simulink model "FaultCheck"  (R2022b)
settings: Solver=FixedStepAuto  StartTime=0.0  StopTime=10  FixedStep=1  RelTol=1e-3
undefined symbols (not defined in the file): C_Flt_IGBTULowerTempConfirmTh_u16, C_Flt_IGBTULowerTempDiagEn_b, C_Flt_IGBTULowerTempErrCode_u16, C_Flt_IGBTULowerTempPowerCoeff, C_Flt_IGBTULowerTempRecoveryTh_u16, C_Flt_IGBTULowerTempRecTh_s32, C_Flt_IGBTULowerTempTrigTh_s32, C_Flt_IGBTUOverTempConfirmTh_u16, C_Flt_IGBTUOverTempDiagEn_b, C_Flt_IGBTUOverTempErrCode_u16, C_Flt_IGBTUOverTempRecoveryTh_u16, C_Flt_IGBTUOverTempRecTh_s32, C_Flt_IGBTUOverTempTrigTh_s32, C_Flt_IGBTVLowerTempConfirmTh_u16, C_Flt_IGBTVLowerTempDiagEn_b, C_Flt_IGBTVLowerTempErrCode_u16, C_Flt_IGBTVLowerTempPowerCoeff, C_Flt_IGBTVLowerTempRecoveryTh_u16, C_Flt_IGBTVLowerTempRecTh_s32, C_Flt_IGBTVLowerTempTrigTh_s32, C_Flt_IGBTVOverTempConfirmTh_u16, C_Flt_IGBTVOverTempDiagEn_b, C_Flt_IGBTVOverTempErrCode_u16, C_Flt_IGBTVOverTempRecoveryTh_u16, C_Flt_IGBTVOverTempRecTh_s32, C_Flt_IGBTVOverTempTrigTh_s32, C_Flt_IGBTWLowerTempConfirmTh_u16, C_Flt_IGBTWLowerTempDiagEn_b, C_Flt_IGBTWLowerTempErrCode_u16, C_Flt_IGBTWLowerTempPowerCoeff, C_Flt_IGBTWLowerTempRecoveryTh_u16, C_Flt_IGBTWLowerTempRecTh_s32, C_Flt_IGBTWLowerTempTrigTh_s32, C_Flt_IGBTWOverTempConfirmTh_u16, C_Flt_IGBTWOverTempDiagEn_b, C_Flt_IGBTWOverTempErrCode_u16, C_Flt_IGBTWOverTempRecoveryTh_u16, C_Flt_IGBTWOverTempRecTh_s32, C_Flt_IGBTWOverTempTrigTh_s32, C_Flt_IuOCConfirmTh_u16, C_Flt_IuOCDiagEn_b, C_Flt_IuOCErrCode_u16, C_Flt_IuOCNegLimit_s32, C_Flt_IuOCPosLimit_s32, C_Flt_IuOCRecoveryTh_u16, C_Flt_IuZeroDriftDiagEn_b, C_Flt_IuZeroDriftErrCode_u16, C_Flt_IvOCConfirmTh_u16, C_Flt_IvOCDiagEn_b, C_Flt_IvOCErrCode_u16, C_Flt_IvOCNegLimit_s32, C_Flt_IvOCPosLimit_s32, C_Flt_IvOCRecoveryTh_u16, C_Flt_IvZeroDriftDiagEn_b, C_Flt_IvZeroDriftErrCode_u16, C_Flt_IwOCConfirmTh_u16, C_Flt_IwOCDiagEn_b, C_Flt_IwOCErrCode_u16, C_Flt_IwOCNegLimit_s32, C_Flt_IwOCPosLimit_s32 ... (+196)
libraries: YS_UserDefined_Library x21, simulink x5
(part 1 of 11)
settings Model: Creator=25313  LastModifiedBy=ZYH
settings OptimizationCC: DefaultParameterBehavior=Inlined  EnhancedBackFolding=on  PassReuseOutputArgsAs=Individual arguments  ZeroExternalMemoryAtStartup=off  ZeroInternalMemoryAtStartup=off  OptimizeBlockOrder=speed  DifferentSizesBufferReuse=on  OptimizationCustomize=off  EfficientTunableParamExpr=on
settings DebuggingCC: ParameterTunabilityLossMsg=error
settings SFSimCC: MATLABDynamicMemAlloc=off
settings RTWCC: Description=Embedded Coder  SystemTargetFile=ert.tlc  GenCodeOnly=on  TemplateMakefile=ert_default_tmf
settings CodeAppCC: ForceParamTrailComments=on  IgnoreCustomStorageClasses=off  OperatorAnnotations=on  SimulinkDataObjDesc=on  SFDataObjDesc=on  InsertBlockDesc=on
settings ERTTargetCC: TargetLangStandard=C99 (ISO)  GenerateSampleERTMain=on  IncludeMdlTerminateFcn=off  RemoveDisableFunc=on  InlinedParameterPlacement=NonHierarchical  ERTCustomFileTemplate=example_file_process.tlc

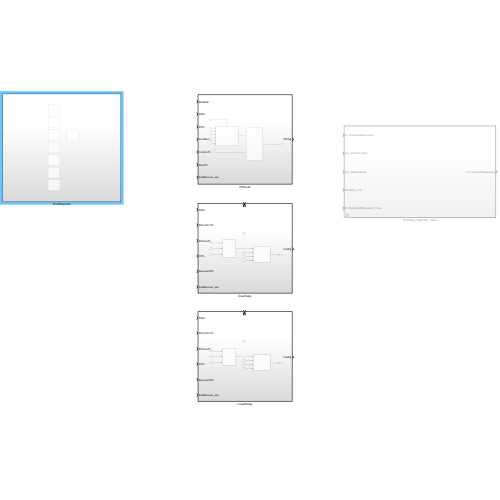
[thumbnail: Simulink's stored preview of the top-level diagram]
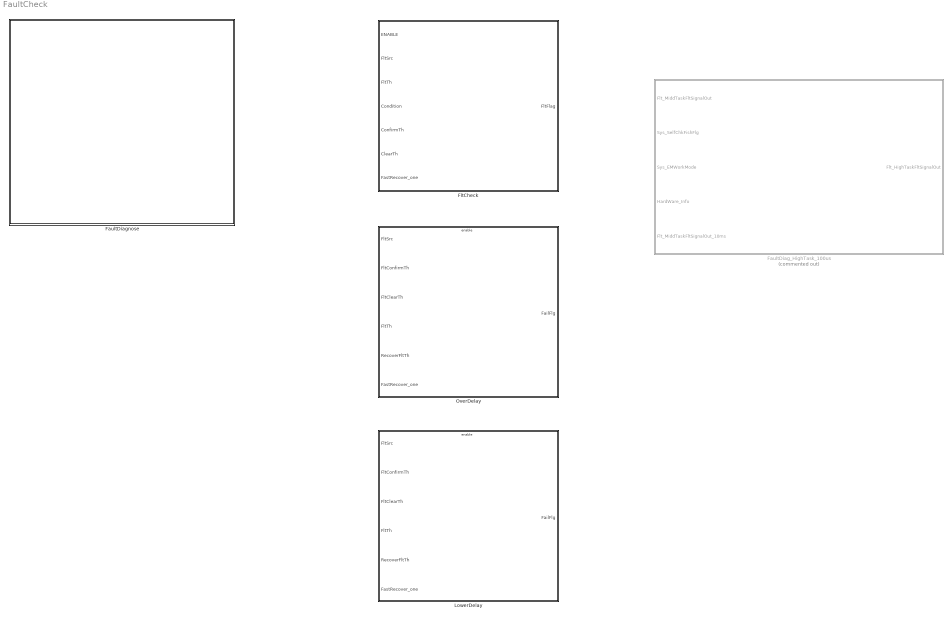
== system FaultCheck ==
  FaultDiag_HighTask_100us : Subsystem  Commented=on  TreatAsAtomicUnit=on  RTWFileName=FaultDiag_HighTask_100us_01
      settings: RTWSystemCode=Nonreusable function  RTWFcnNameOpts=Use subsystem name  RTWFileNameOpts=User specified
  FaultDiagnose : Subsystem
  FltCheck : Subsystem  TreatAsAtomicUnit=on
  LowerDelay : Subsystem
  OverDelay : Subsystem

== system FaultCheck/FaultDiag_HighTask_100us ==
  note: 其诊断主要包括：
      | 1、三相软件过流诊断
      | 2、硬件过流诊断
      | 3、电流零飘诊断
      | 4、母线电压诊断（包括一级和二级过压、欠压诊断）
      | 5、驱动电压诊断
      | 6、驱动上桥诊断
      | 7、驱动下桥诊断
      | 8、旋变电压诊断
      | 9、旋变信号诊断
      | 10、硬件电压诊断
  note: 高频故障诊断主要包括以下几个模块：
      |
      | 信号输入
      |
      | 故障诊断
      |
      | 故障收集（高频故障仲裁）
      |
      | 故障仲裁
      |
      | 信号输出
  Flt_MiddTaskFltSignalOut : Inport
  Sys_SelfChkFishFlg : Inport  Port=2
  Sys_EMWorkMode : Inport  Port=3
  HardWare_Info : Inport  Port=4
  Flt_MiddTaskFltSignalOut_10ms : Inport  Port=5
  FltDetermine : Subsystem
  FltDetn : Subsystem
  FltHandle : Subsystem
  SignalInput1 : Subsystem
  SignalOutput : Subsystem
  Flt_HighTaskFltSignalOut : Outport
  wires:
  Flt_MiddTaskFltSignalOut/1 -> SignalInput1/4(Flt_MiddTaskFltSignalOut)
  SignalInput1/1(FltSignalBus) -> FltDetn/1(FltSignalInput), [FltSignalBus]
  FltDetn/1(FltDetnOut) -> FltHandle/2(DltDetnOut)
  SignalOutput/1(Flt_HighTaskFltSignalOut) -> Flt_HighTaskFltSignalOut/1
  Sys_SelfChkFishFlg/1 -> SignalInput1/2(Sys_SelfChkFishFlg)
  Sys_EMWorkMode/1 -> SignalInput1/3(Sys_EMWorkMode)
  [FltSignalBus] -> FltHandle/1(FltSignalBus)
  FltHandle/1(FltHandleOut) -> FltDetermine/1(FltHandleOut)
  [FltSignalBus] -> FltDetermine/2(FltSignalBus)
  FltDetermine/1(FltDetermineOut) -> SignalOutput/1(FltDetermineOut)
  HardWare_Info/1 -> SignalInput1/1(HardWare_Info)
  Flt_MiddTaskFltSignalOut_10ms/1 -> SignalInput1/5(Flt_MiddTaskFltSignalOut_10ms)

== system FaultCheck/FaultDiagnose ==
  CurrZeroDriftFltDiag : Subsystem
  IGBTTempDiag : Subsystem
  MotorSpdFltDiag : Subsystem
  MotorTempDiag : Subsystem
  PCBTempDiag : Subsystem
  PhaseCurrDiag : Subsystem  TreatAsAtomicUnit=on
  UdcLowerOneDiag : Subsystem
  UdcLowerTwoDiag : Subsystem
  UdcOverOneDiag : Subsystem
  UdcOverTwoDiag : Subsystem

== system FaultCheck/FltCheck ==
  ENABLE : Inport
  FltSrc : Inport  Port=2
  FltTh : Inport  Port=3
  Condition : Inport  Port=4
  ConfirmTh : Inport  Port=5
  ClearTh : Inport  Port=6
  FastRecover_one : Inport  Port=7
  Chart : Stateflow chart  TreatAsAtomicUnit=on
  Determination : Subsystem
  FltFlag : Outport
  wires:
  Chart/1(FltFlag) -> FltFlag/1
  FltSrc/1 -> Determination/1(FltSrc)
  FastRecover_one/1 -> Chart/2(FastRecover_one), Determination/6(FastRecover_one)
  Determination/1(FltConfirmed) -> Chart/1(FltConfirmed)
  ConfirmTh/1 -> Determination/4(ConfirmTh)
  ENABLE/1 -> Determination/Enable
  ClearTh/1 -> Determination/5(ClearTh)
  FltTh/1 -> Determination/2(FltTh)
  Condition/1 -> Determination/3(Condition)

== system FaultCheck/LowerDelay ==
  FltSrc : Inport
  FltConfirmTh : Inport  Port=2
  FltClearTh : Inport  Port=3
  FltTh : Inport  Port=4
  RecoverFltTh : Inport  Port=5
  FastRecover_one : Inport  Port=6
  Enable : EnablePort
  Hysteresis : Subsystem
  Relay : Subsystem
  FailFlg : Outport
  wires:
  FltTh/1 -> Relay/2(FltTh)
  Hysteresis/1(Out) -> FailFlg/1
  RecoverFltTh/1 -> Relay/3(RecoverFltTh)
  FastRecover_one/1 -> Hysteresis/4(FastRecover_one)
  FltSrc/1 -> Relay/1(FltSrc)
  FltClearTh/1 -> Hysteresis/3(ClearTh)
  Relay/1(Fail) -> Hysteresis/1(Fail)
  FltConfirmTh/1 -> Hysteresis/2(ConfirmTh)

== system FaultCheck/OverDelay ==
  FltSrc : Inport
  FltConfirmTh : Inport  Port=2
  FltClearTh : Inport  Port=3
  FltTh : Inport  Port=4
  RecoverFltTh : Inport  Port=5
  FastRecover_one : Inport  Port=6
  Enable : EnablePort
  Hysteresis : Subsystem
  Relay : Subsystem
  FailFlg : Outport
  wires:
  FltConfirmTh/1 -> Hysteresis/2(ConfirmTh)
  Relay/1(Fail) -> Hysteresis/1(Fail)
  FltClearTh/1 -> Hysteresis/3(ClearTh)
  FltSrc/1 -> Relay/1(FltSrc)
  FastRecover_one/1 -> Hysteresis/4(FastRecover_one)
  RecoverFltTh/1 -> Relay/3(RecoverFltTh)
  Hysteresis/1(Out) -> FailFlg/1
  FltTh/1 -> Relay/2(FltTh)

== system FaultCheck/FaultDiag_HighTask_100us/FltDetermine ==
  note: 整个故障诊断的仲裁模块，选择高频，中频和低频三种故障诊断周期的最大故障等级，最小降功率系数输出
  FltHandleOut : Inport
  FltSignalBus : Inport  Port=2
  Bus Creator : BusCreator  Inputs=4
  Bus Selector : BusSelector  OutputSignals=Flt_HighTaskFltSignalOut.Flt_HighTaskFltLvlOut_100us,Flt_HighTaskFltSignalOut.Flt_HighTaskPowRecCoef_100us
  Bus Selector1 : BusSelector  OutputSignals=Flt_FltLvlOut_1ms,Flt_PowRecCoef_1ms,Flt_MiddTaskFltLvl_10ms,Flt_MiddTaskPowRecCoef_10ms
  FliLvlOut : Subsystem
  PowRecCoefOut : Subsystem
  Subsystem1 : Subsystem
  FltDetermineOut : Outport
  wires:
  FliLvlOut/1(Flt_FltLvlOut) -> [Flt_FltLvlOut], Bus Creator/2  "Flt_FltLvlOut"
  PowRecCoefOut/1(Flt_PowRecCoef) -> Bus Creator/3  "Flt_PowRecCoefOut"
  Subsystem1/1(Flt_SwtForFOC) -> Bus Creator/4  "Flt_SwtForFOC"
  FltHandleOut/1 -> Bus Selector/1, [FltHandleOut]
  FltSignalBus/1 -> Bus Selector1/1
  Bus Creator/1 -> FltDetermineOut/1
  Bus Selector/1 -> [Flt_HighTaskFltLvlOut]  "<Flt_HighTaskFltLvlOut_100us>"
  Bus Selector/2 -> [Flt_HighTaskPowRecCoef]  "<Flt_HighTaskPowRecCoef_100us>"
  Bus Selector1/1 -> [Flt_MiddTaskFltLvlOut]  "<Flt_FltLvlOut_1ms>"
  Bus Selector1/2 -> [Flt_MiddTaskPowRecCoef]  "<Flt_PowRecCoef_1ms>"
  [Flt_HighTaskFltLvlOut] -> FliLvlOut/1(Flt_HighTaskFltLvlOut)
  [Flt_LowTaskFltLvlOut] -> FliLvlOut/3(Flt_LowTaskFltLvlOut)
  [Flt_LowTaskPowRecCoef] -> PowRecCoefOut/3(Flt_LowTaskPowRecCoef)
  [Flt_FltLvlOut] -> Subsystem1/1(Flt_FltLvlOut)
  [FltHandleOut] -> Bus Creator/1  "FltHandleOut"
  [Flt_HighTaskPowRecCoef] -> PowRecCoefOut/1(Flt_HighTaskPowRecCoef)
  Bus Selector1/4 -> [Flt_LowTaskPowRecCoef]  "<Flt_MiddTaskPowRecCoef_10ms>"
  Bus Selector1/3 -> [Flt_LowTaskFltLvlOut]  "<Flt_MiddTaskFltLvl_10ms>"
  [Flt_MiddTaskFltLvlOut] -> FliLvlOut/2(Flt_MiddTaskFltLvlOut)
  [Flt_MiddTaskPowRecCoef] -> PowRecCoefOut/2(Flt_MiddTaskPowRecCoef)

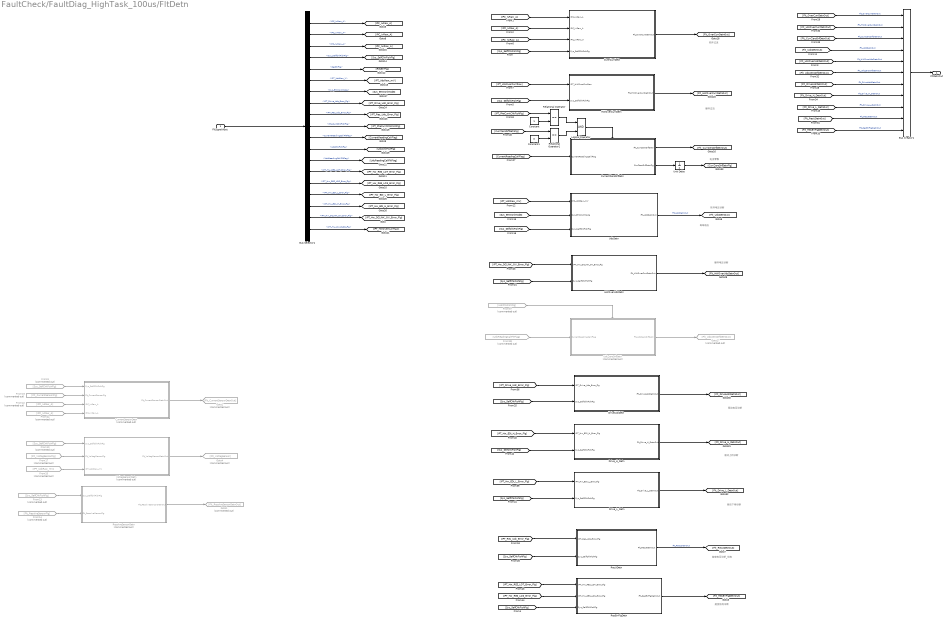
== system FaultCheck/FaultDiag_HighTask_100us/FltDetn ==
  note: 软件过流
  note: 旋变信号诊断
  note: 母线电压
  note: 旋变电压诊断_供电
  note: 硬件过流
  note: 电流零飘
  note: 软件电压诊断
  note: 硬件电压诊断
  note: 驱动电压诊断
  note: 驱动上桥诊断
  note: 驱动下桥诊断
  FltSignalInput : Inport
  Bus Creator1 : BusCreator  Inputs=11
  Bus Selector1 : BusSelector  OutputSignals=IPC_IuRaw_A,IPC_IvRaw_A,IPC_IwRaw_A,Sys_SelfChkFishFlg,ResErrFlg,IPT_UdcRaw_V,Sys_EMWorkMode,HardwareFault_Info.IPT_Drive_Udc_Error_Flg,HardwareFault_Info.IPT_Res_Udc_Error_Flg,HardwareFault_Info.PhaCurrtChkFishFlg,HardwareFault_Info.CurrentReadingCaliFltFlag,HardwareFault_Info.UdcChkFishFlg,HardwareFault_Info.UdcReadingCaliFltFlag,HardwareFault_Info.IPT_Hw_RES_LOT_Error_Flg,HardwareFault_Info.IPT_Hw_RES_LOS_Error_Flg,HardwareFault_Info.IPT_Hw_EDI_L_Error_Flg,HardwareFault_Info.IPT_Hw_EDI_H_Error_Flg,HardwareFault_Info.IPT_Hw_DCLINK_OV_Error_Flg,HardwareFault_Info.IPT_Hw_OV_CURR_Flg
  Constant : Constant  OutDataTypeStr=uint8
  Constant1 : Constant  Value=0  OutDataTypeStr=uint8
  CurrentSensorDetn : Subsystem  Commented=on
  CurrentZeroDrfDetn : Subsystem
  DriveUdcDetn : Subsystem
  Drive_H_Detn : Subsystem
  Drive_L_Detn : Subsystem
  From10 : From  Commented=on  GotoTag=Sys_SelfChkFishFlg
  From13 : From  Commented=on  GotoTag=Sys_SelfChkFishFlg
  From14 : From  Commented=on  GotoTag=Flt_ResolveSensorFlg
  From17 : From  Commented=on  GotoTag=Flt_VoltagSensorFlg
  From19 : From  Commented=on  GotoTag=Flt_CurrentSensorFlg
  From20 : From  Commented=on  GotoTag=IPT_UdcRaw_mV
  From22 : From  Commented=on  GotoTag=IPC_IuRaw_A
  From24 : From  Commented=on  GotoTag=IPC_IvRaw_A
  From37 : From  Commented=on  GotoTag=UdcChkFishFlg
  From38 : From  Commented=on  GotoTag=UdcReadingCaliFltFlag
  From9 : From  Commented=on  GotoTag=Sys_SelfChkFishFlg
  Goto1 : Goto  Commented=on  GotoTag=Flt_ResolveSensorDetnOut
  Goto2 : Goto  Commented=on  GotoTag=Flt_CurrentSensorDetnOut
  Goto27 : Goto  Commented=on  GotoTag=Flt_UdcZeroDrfDetnOut
  Goto4 : Goto  Commented=on  GotoTag=Flt_VoltagSensor
  HWOverCurrDetn : Subsystem
  HWOverUdcDetn : Subsystem
  Logical Operator : Logic  AllPortsSameDT=off  OutDataTypeStr=boolean
  OverCurrDetn : Subsystem
  RecUDetn : Subsystem
  Relational Operator : RelationalOperator  Operator===  OutDataTypeStr=boolean  RndMeth=Simplest  InputSameDT=off
  Relational Operator1 : RelationalOperator  Operator===  OutDataTypeStr=boolean  RndMeth=Simplest  InputSameDT=off
  ResErrFlgDetn : Subsystem
  ResolveSensorDetn : Subsystem  Commented=on
  UdcDetn : Subsystem
  UdcZeroDrfDetn : Subsystem  Commented=on
  Unit Delay : UnitDelay  SampleTime=-1  HasFrameUpgradeWarning=on
  VoltagSensorDetn : Subsystem  Commented=on
  FltDetnOut : Outport
  wires:
  [Sys_SelfChkFishFlg] -> OverCurrDetn/4(Sys_SelfChkFishFlg)
  [IPC_IuRaw_A] -> OverCurrDetn/1(IPC_IuRaw_A)
  [IPC_IvRaw_A] -> OverCurrDetn/2(IPC_IvRaw_A)
  OverCurrDetn/1(Flt_OverCurrDetnOut) -> [Flt_OverCurrDetnOut]
  [IPT_HWOverCurrRaw] -> HWOverCurrDetn/1(IPT_HWOverCurrRaw)
  HWOverCurrDetn/1(Flt_HWOverCurrDetnOut) -> [Flt_HWOverCurrDetnOut]
  [CurrentReadingCaliFlag] -> CurrentZeroDrfDetn/1(CurrentReadingCaliFlag)
  CurrentZeroDrfDetn/1(Flt_CurrZeroDrfDetn) -> [Flt_CurrZeroDrfDetnOut]
  [IPT_Hw_RES_LOT_Error_Flg] -> ResErrFlgDetn/1(IPT_Hw_RES_LOT_Error_Flg)
  [Sys_SelfChkFishFlg] -> ResErrFlgDetn/3(Sys_SelfChkFishFlg)
  [Sys_SelfChkFishFlg] -> HWOverCurrDetn/2(Sys_SelfChkFishFlg)
  ResErrFlgDetn/1(Flt_ResErrFlgDetnOut) -> [Flt_ResErrFlgDetnOut]
  FltSignalInput/1 -> Bus Selector1/1
  Bus Selector1/5 -> [ResErrFlg]  "<ResErrFlg>"
  Bus Selector1/2 -> [IPC_IvRaw_A]  "<IPC_IvRaw_A>"
  Bus Selector1/4 -> [Sys_SelfChkFishFlg]  "<Sys_SelfChkFishFlg>"
  Bus Selector1/17 -> [IPT_Hw_EDI_H_Error_Flg]  "<IPT_Hw_EDI_H_Error_Flg>"
  Bus Selector1/18 -> [IPT_Hw_DCLINK_OV_Error_Flg]  "<IPT_Hw_DCLINK_OV_Error_Flg>"
  Bus Selector1/6 -> [IPT_UdcRaw_mV]  "<IPT_UdcRaw_V>"
  Bus Selector1/1 -> [IPC_IuRaw_A]  "<IPC_IuRaw_A>"
  [Sys_EMWorkMode] -> UdcDetn/2(Sys_EMWorkMode)
  From13/1 -> ResolveSensorDetn/1(Sys_SelfChkFishFlg)
  From14/1 -> ResolveSensorDetn/2(Flt_ResolveSensorFlg)
  [IPT_UdcRaw_mV] -> UdcDetn/1(IPC_UdcRaw_mV)
  [IPT_Res_Udc_Error_Flg] -> RecUDetn/1(IPT_Res_Udc_Error_Flg)
  From19/1 -> CurrentSensorDetn/2(Flt_CurrentSensorFlg)
  From22/1 -> CurrentSensorDetn/3(IPC_IuRaw_A)
  VoltagSensorDetn/1(Flt_VoltagSensorDetnOut) -> Goto4/1
  From9/1 -> CurrentSensorDetn/1(Sys_SelfChkFishFlg)
  From20/1 -> VoltagSensorDetn/3(IPT_UdcRaw_mV)
  [Sys_SelfChkFishFlg] -> RecUDetn/2(Sys_SelfChkFishFlg)
  CurrentSensorDetn/1(Flt_CurrentSensorDetnOut) -> Goto2/1
  From10/1 -> VoltagSensorDetn/1(Sys_SelfChkFishFlg)
  RecUDetn/1(Flt_RecUDetnOut) -> [Flt_RecUDetnOut]  "Flt_RecUDetnOut"
  From24/1 -> CurrentSensorDetn/4(IPC_IvRaw_A)
  From17/1 -> VoltagSensorDetn/2(Flt_VoltagSensorFlg)
  [Sys_SelfChkFishFlg] -> UdcDetn/3(Sys_SelfChkFishFlg)
  UdcDetn/1(Flt_UdcDetnOut) -> [Flt_UdcDetnOut]  "Flt_UdcDetnOut"
  ResolveSensorDetn/1(Flt_ResolveSensorDetnOut) -> Goto1/1
  [Flt_RecUDetnOut] -> Bus Creator1/10  "Flt_RecUDetnOut"
  Bus Creator1/1 -> FltDetnOut/1
  [Flt_ResErrFlgDetnOut] -> Bus Creator1/11  "Flt_ResErrFlgDetnOut"
  [Flt_HWOverCurrDetnOut] -> Bus Creator1/2  "Flt_HWOverCurrDetnOut"
  [Flt_UdcDetnOut] -> Bus Creator1/4  "Flt_UdcDetnOut"
  [Flt_CurrZeroDrfDetnOut] -> Bus Creator1/3  "Flt_CurrZeroDrfDetnOut"
  [Flt_OverCurrDetnOut] -> Bus Creator1/1  "Flt_OverCurrDetnOut"
  Bus Selector1/3 -> [IPC_IwRaw_A]  "<IPC_IwRaw_A>"
  [IPC_IwRaw_A] -> OverCurrDetn/3(IPC_IwRaw_A)
  Bus Selector1/7 -> [Sys_EMWorkMode]  "<Sys_EMWorkMode>"
  Bus Selector1/8 -> [IPT_Drive_Udc_Error_Flg]  "<IPT_Drive_Udc_Error_Flg>"
  Bus Selector1/9 -> [IPT_Res_Udc_Error_Flg]  "<IPT_Res_Udc_Error_Flg>"
  Bus Selector1/11 -> [CurrentReadingCaliFlag]  "<CurrentReadingCaliFltFlag>"
  Bus Selector1/13 -> [UdcReadingCaliFltFlag]  "<UdcReadingCaliFltFlag>"
  Bus Selector1/14 -> [IPT_Hw_RES_LOT_Error_Flg]  "<IPT_Hw_RES_LOT_Error_Flg>"
  Bus Selector1/15 -> [IPT_Hw_RES_LOS_Error_Flg]  "<IPT_Hw_RES_LOS_Error_Flg>"
  Bus Selector1/16 -> [IPT_Hw_EDI_L_Error_Flg]  "<IPT_Hw_EDI_L_Error_Flg>"
  Bus Selector1/19 -> [IPT_HWOverCurrRaw]  "<IPT_Hw_OV_CURR_Flg>"
  [Sys_SelfChkFishFlg] -> HWOverUdcDetn/2(Sys_SelfChkFishFlg)
  [IPT_Hw_DCLINK_OV_Error_Flg] -> HWOverUdcDetn/1(IPT_Hw_DCLINK_OV_Error_Flg)
  UdcZeroDrfDetn/1(Flt_UdcZeroDrfDetn) -> Goto27/1
  From38/1 -> UdcZeroDrfDetn/1(CurrentReadingCaliFlag)
  From37/1 -> UdcZeroDrfDetn/Trigger
  HWOverUdcDetn/1(Flt_HWOverCurrDetnOut) -> [Flt_HWOverUdcDetnOut]
  Bus Selector1/10 -> [IPT_PhaCurrtChkFishFlg]  "<PhaCurrtChkFishFlg>"
  Bus Selector1/12 -> [UdcChkFishFlg]  "<UdcChkFishFlg>"
  DriveUdcDetn/1(Flt_DriveUdcDetnOut) -> [Flt_DriveUdcDetnOut]
  [IPT_Drive_Udc_Error_Flg] -> DriveUdcDetn/1(IPT_Drive_Udc_Error_Flg)
  [Sys_SelfChkFishFlg] -> DriveUdcDetn/2(Sys_SelfChkFishFlg)
  [IPT_Hw_EDI_L_Error_Flg] -> Drive_L_Detn/1(IPT_Hw_EDI_L_Error_Flg)
  [IPT_Hw_EDI_H_Error_Flg] -> Drive_H_Detn/1(IPT_Hw_EDI_H_Error_Flg)
  [Sys_SelfChkFishFlg] -> Drive_H_Detn/2(Sys_SelfChkFishFlg)
  [Sys_SelfChkFishFlg] -> Drive_L_Detn/2(Sys_SelfChkFishFlg)
  [IPT_Hw_RES_LOS_Error_Flg] -> ResErrFlgDetn/2(IPT_Hw_RES_LOS_Error_Flg)
  [Flt_HWOverUdcDetnOut] -> Bus Creator1/5  "Flt_HWOverUdcDetnOut"
  [Flt_UdcZeroDrfDetnOut] -> Bus Creator1/6  "Flt_UdcZeroDrfDetnOut"
  Drive_L_Detn/1(Flt_Drive_L_DetnOut) -> [Flt_Drive_L_DetnOut]
  Drive_H_Detn/1(Flt_Drive_H_DetnOut) -> [Flt_Drive_H_DetnOut]
  [Flt_DriveUdcDetnOut] -> Bus Creator1/7  "Flt_DriveUdcDetnOut"
  [Flt_Drive_H_DetnOut] -> Bus Creator1/8  "Flt_Drive_H_DetnOut"
  [Flt_Drive_L_DetnOut] -> Bus Creator1/9  "Flt_Drive_L_DetnOut"
  CurrentZeroDrfDetn/2(CurrZeroDrfDetnFlg) -> Unit Delay/1
  [IPT_PhaCurrtChkFishFlg] -> Relational Operator/1
  Relational Operator/1 -> Logical Operator/1
  [CurrZeroDrfDetnFlg] -> Relational Operator1/1
  Constant/1 -> Relational Operator/2
  Constant1/1 -> Relational Operator1/2
  Relational Operator1/1 -> Logical Operator/2
  Logical Operator/1 -> CurrentZeroDrfDetn/Enable
  Unit Delay/1 -> [CurrZeroDrfDetnFlg]

== system FaultCheck/FaultDiag_HighTask_100us/FltHandle ==
  note: 中频故障诊断的故障仲裁部分，选择故障等级最高的和故障降功率系数最低的输出，以应付多故障同时发生的情况
  FltSignalBus : Inport
  DltDetnOut : Inport  Port=2
  Bus Creator : BusCreator  Inputs=2
  Bus Creator1 : BusCreator  Inputs=3
  Bus Creator2 : BusCreator  Inputs=2
  FltLvl : Subsystem
  PowRecCoef : Subsystem
  ValOut : Subsystem
  FltHandleOut : Outport
  wires:
  Bus Creator/1 -> Bus Creator2/2  "Flt_HighTaskFltSignalOut"
  DltDetnOut/1 -> PowRecCoef/1(FltDetnIn), FltLvl/1(FltDetnIn)
  FltLvl/1(Flt_HighTaskFltLvlOut) -> Bus Creator/1  "Flt_HighTaskFltLvlOut_100us"
  PowRecCoef/1(Flt_HighTaskPowRecCoef) -> Bus Creator/2  "Flt_HighTaskPowRecCoef_100us"
  FltSignalBus/1 -> ValOut/1(FltSignalBus)
  ValOut/1(Flt_IuOut_A) -> Bus Creator1/1  "IPC_IuRaw_A"
  ValOut/2(Flt_IvOut_A) -> Bus Creator1/2  "IPC_IvRaw_A"
  Bus Creator2/1 -> FltHandleOut/1
  Bus Creator1/1 -> Bus Creator2/1  "Flt_HighTaskSignalOut"
  ValOut/3(Flt_IwOut_A) -> Bus Creator1/3  "IPC_IwRaw_A"

== system FaultCheck/FaultDiag_HighTask_100us/SignalInput1 ==
  HardWare_Info : Inport
  Sys_SelfChkFishFlg : Inport  Port=2
  Sys_EMWorkMode : Inport  Port=3
  Flt_MiddTaskFltSignalOut : Inport  Port=4
  Flt_MiddTaskFltSignalOut_10ms : Inport  Port=5
  Bus Creator : BusCreator  Inputs=14
  Bus Selector : BusSelector  OutputSignals=IPT_IRaw_A.IPC_IuRaw_A,IPT_IRaw_A.IPC_IvRaw_A,IPT_IRaw_A.IPC_IwRaw_A,ResErrFlg,IPT_TempRaw_degC.IPT_PCBTempRaw_degC,IPT_TempRaw_degC.IPT_MotorTempLow_degC_Meas,IPT_UdcRaw_V,HardwareFault_Info
  Bus Selector1 : BusSelector  OutputSignals=Flt_PowRecCoef_1ms,Flt_FltLvlOut_1ms
  Bus Selector2 : BusSelector  OutputSignals=Flt_MiddTaskFltLvl_10ms,Flt_MiddTaskPowRecCoef_10ms
  FltSignalBus : Outport
  wires:
  Bus Selector1/2 -> Bus Creator/12  "<Flt_FltLvlOut_1ms>"
  Bus Selector1/1 -> Bus Creator/11  "<Flt_PowRecCoef_1ms>"
  Sys_EMWorkMode/1 -> Bus Creator/10  "Sys_EMWorkMode"
  Sys_SelfChkFishFlg/1 -> Bus Creator/9  "Sys_SelfChkFishFlg"
  Flt_MiddTaskFltSignalOut/1 -> Bus Selector1/1
  HardWare_Info/1 -> Bus Selector/1
  Bus Creator/1 -> FltSignalBus/1
  Flt_MiddTaskFltSignalOut_10ms/1 -> Bus Selector2/1
  Bus Selector2/1 -> Bus Creator/13  "<Flt_MiddTaskFltLvl_10ms>"
  Bus Selector2/2 -> Bus Creator/14  "<Flt_MiddTaskPowRecCoef_10ms>"
  Bus Selector/1 -> Bus Creator/1  "<IPC_IuRaw_A>"
  Bus Selector/2 -> Bus Creator/2  "<IPC_IvRaw_A>"
  Bus Selector/3 -> Bus Creator/3  "<IPC_IwRaw_A>"
  Bus Selector/4 -> Bus Creator/4  "<ResErrFlg>"
  Bus Selector/5 -> Bus Creator/5  "<IPT_PCBTempRaw_degC>"
  Bus Selector/6 -> Bus Creator/6  "<IPT_MotorTempLow_degC_Meas>"
  Bus Selector/7 -> Bus Creator/7  "<IPT_UdcRaw_V>"
  Bus Selector/8 -> Bus Creator/8  "<HardwareFault_Info>"

== system FaultCheck/FaultDiag_HighTask_100us/SignalOutput ==
  FltDetermineOut : Inport
  Bus Creator : BusCreator  Inputs=6
  Bus Selector : BusSelector  OutputSignals=FltHandleOut.Flt_HighTaskSignalOut.IPC_IuRaw_A,FltHandleOut.Flt_HighTaskSignalOut.IPC_IvRaw_A,FltHandleOut.Flt_HighTaskSignalOut.IPC_IwRaw_A,Flt_PowRecCoefOut,Flt_FltLvlOut,Flt_SwtForFOC
  Constant : Constant  OutDataTypeStr=uint8
  Gain{,1..2,4} (4 alike) : Gain  OutDataTypeStr=single
  Product : Product  OutDataTypeStr=uint8
  Flt_HighTaskFltSignalOut : Outport
  wires:
  Bus Creator/1 -> Flt_HighTaskFltSignalOut/1
  FltDetermineOut/1 -> Bus Selector/1
  Bus Selector/1 -> Gain/1  "<IPC_IuRaw_A>"
  Bus Selector/2 -> Gain1/1  "<IPC_IvRaw_A>"
  Bus Selector/4 -> Gain2/1  "<Flt_PowRecCoefOut>"
  Bus Selector/6 -> Bus Creator/6  "<Flt_SwtForFOC>"
  Gain/1 -> Bus Creator/1  "IPC_luRaw_A1"
  Gain1/1 -> Bus Creator/2  "IPC_IvRaw_A1"
  Gain2/1 -> Bus Creator/4  "Flt_PowRecCoefOut1"
  Bus Selector/3 -> Gain4/1  "<IPC_IwRaw_A>"
  Gain4/1 -> Bus Creator/3  "IPC_IwRaw_A1"
  Bus Selector/5 -> Product/1  "<Flt_FltLvlOut>"
  Product/1 -> Bus Creator/5  "Flt_FltLvlOut1"
  Constant/1 -> Product/2

== system FaultCheck/FaultDiagnose/CurrZeroDriftFltDiag ==
  SysSelfCheckDownFlg : Inport
  IuZeroDriftFltFlg : Inport  Port=2
  IvZeroDriftFltFlg : Inport  Port=3
  IwZeroDriftFltFlg : Inport  Port=4
  Bus Creator : BusCreator  Inputs=3
  IuZeroDriftDiag : Subsystem
  IvZeroDriftDiag : Subsystem
  IwZeroDriftDiag : Subsystem
  Logical Operator : Logic  Operator=NOT  AllPortsSameDT=off  OutDataTypeStr=boolean
  Logical Operator1 : Logic  Operator=NOT  AllPortsSameDT=off  OutDataTypeStr=boolean
  Logical Operator2 : Logic  Operator=NOT  AllPortsSameDT=off  OutDataTypeStr=boolean
  Unit Delay : UnitDelay  SampleTime=-1  HasFrameUpgradeWarning=on
  Unit Delay1 : UnitDelay  SampleTime=-1  HasFrameUpgradeWarning=on
  Unit Delay2 : UnitDelay  SampleTime=-1  HasFrameUpgradeWarning=on
  PhaseCurrZeroDriftFltInfo : Outport
  wires:
  IuZeroDriftFltFlg/1 -> IuZeroDriftDiag/2(IuZeroDriftFltFlg)
  IuZeroDriftDiag/1(IuZeroDriftDiagDownFlg) -> Unit Delay/1
  Logical Operator/1 -> IuZeroDriftDiag/Enable
  Unit Delay/1 -> Logical Operator/1
  IvZeroDriftFltFlg/1 -> IvZeroDriftDiag/2(IvZeroDriftFltFlg)
  Unit Delay1/1 -> Logical Operator1/1
  Logical Operator1/1 -> IvZeroDriftDiag/Enable
  IvZeroDriftDiag/1(IvZeroDriftDiagDownFlg) -> Unit Delay1/1
  IwZeroDriftFltFlg/1 -> IwZeroDriftDiag/2(IwZeroDriftFltFlg)
  Unit Delay2/1 -> Logical Operator2/1
  Logical Operator2/1 -> IwZeroDriftDiag/Enable
  IwZeroDriftDiag/1(IwZeroDriftDiagDownFlg) -> Unit Delay2/1
  IuZeroDriftDiag/2(IuZeroDriftFltInfo) -> Bus Creator/1  "IuZeroDriftFltInfo"
  IvZeroDriftDiag/2(IvZeroDriftFltInfo) -> Bus Creator/2  "IvZeroDriftFltInfo"
  IwZeroDriftDiag/2(IwZeroDriftFltInfo) -> Bus Creator/3  "IwZeroDriftFltInfo"
  Bus Creator/1 -> PhaseCurrZeroDriftFltInfo/1
  SysSelfCheckDownFlg/1 -> IwZeroDriftDiag/1(SysSelfCheckDownFlg), IvZeroDriftDiag/1(SysSelfCheckDownFlg), IuZeroDriftDiag/1(SysSelfCheckDownFlg)

== system FaultCheck/FaultDiagnose/IGBTTempDiag ==
  SysSelfCheckDownFlg : Inport
  IGBTUTemp : Inport  Port=2
  IGBTVTemp : Inport  Port=3
  IGBTWTemp : Inport  Port=4
  Bus Creator : BusCreator  Inputs=6
  IGBTULowerTempDiag : Subsystem
  IGBTUOverTempDiag : Subsystem
  IGBTVLowerTempDiag : Subsystem
  IGBTVOverTempDiag : Subsystem
  IGBTWLowerTempDiag : Subsystem
  IGBTWOverTempDiag : Subsystem
  IGBTTempFltInfo : Outport
  wires:
  SysSelfCheckDownFlg/1 -> IGBTWOverTempDiag/1(SysSelfCheckDownFlg), IGBTWLowerTempDiag/1(SysSelfCheckDownFlg), IGBTVLowerTempDiag/1(SysSelfCheckDownFlg), IGBTVOverTempDiag/1(SysSelfCheckDownFlg), IGBTULowerTempDiag/1(SysSelfCheckDownFlg), IGBTUOverTempDiag/1(SysSelfCheckDownFlg)
  IGBTUTemp/1 -> IGBTULowerTempDiag/2(IGBTUTemp), IGBTUOverTempDiag/2(IGBTUTemp)
  IGBTVTemp/1 -> IGBTVLowerTempDiag/2(IGBTVTemp), IGBTVOverTempDiag/2(IGBTVTemp)
  IGBTWTemp/1 -> IGBTWLowerTempDiag/2(IGBTWTemp), IGBTWOverTempDiag/2(IGBTWTemp)
  IGBTULowerTempDiag/1(IGBTULowerTempFltInfo) -> Bus Creator/2  "IGBTULowerTempFltInfo"
  IGBTUOverTempDiag/1(IGBTUOverTempFltInfo) -> Bus Creator/1  "IGBTUOverTempFltInfo"
  IGBTVOverTempDiag/1(IGBTVOverTempFltInfo) -> Bus Creator/3  "IGBTVOverTempFltInfo"
  IGBTVLowerTempDiag/1(IGBTVLowerTempFltInfo) -> Bus Creator/4  "IGBTVLowerTempFltInfo"
  IGBTWOverTempDiag/1(IGBTWOverTempFltInfo) -> Bus Creator/5  "IGBTWOverTempFltInfo"
  IGBTWLowerTempDiag/1(IGBTWLowerTempFltInfo) -> Bus Creator/6  "IGBTWLowerTempFltInfo"
  Bus Creator/1 -> IGBTTempFltInfo/1

== system FaultCheck/FaultDiagnose/MotorSpdFltDiag ==
  SysSelfCheckDownFlg : Inport
  MotorSpd : Inport  Port=2
  Bus Creator : BusCreator  Inputs=4
  MotorOverSpdOneNegDiag : Subsystem
  MotorOverSpdOnePosDiag : Subsystem
  MotorOverSpdTwoNegDiag : Subsystem
  MotorOverSpdTwoPosDiag : Subsystem
  PCBTempFltInfo : Outport
  wires:
  Bus Creator/1 -> PCBTempFltInfo/1
  MotorOverSpdOneNegDiag/1(MotorOverSpdOneNegFltInfo) -> Bus Creator/2  "MotorOverSpdOneNegFltInfo"
  SysSelfCheckDownFlg/1 -> MotorOverSpdTwoNegDiag/1(SysSelfCheckDownFlg), MotorOverSpdTwoPosDiag/1(SysSelfCheckDownFlg), MotorOverSpdOneNegDiag/1(SysSelfCheckDownFlg), MotorOverSpdOnePosDiag/1(SysSelfCheckDownFlg)
  MotorSpd/1 -> MotorOverSpdTwoNegDiag/2(MotorSpd), MotorOverSpdTwoPosDiag/2(MotorSpd), MotorOverSpdOneNegDiag/2(MotorSpd), MotorOverSpdOnePosDiag/2(MotorSpd)
  MotorOverSpdOnePosDiag/1(MotorOverSpdOnePosFltInfo) -> Bus Creator/1  "MotorOverSpdOnePosFltInfo"
  MotorOverSpdTwoPosDiag/1(MotorOverSpdTwoPosFltInfo) -> Bus Creator/3  "MotorOverSpdOnePosFltInfo"
  MotorOverSpdTwoNegDiag/1(MotorOverSpdTwoNegFltInfo) -> Bus Creator/4  "MotorOverSpdOneNegFltInfo"

== system FaultCheck/FaultDiagnose/MotorTempDiag ==
  SysSelfCheckDownFlg : Inport
  MotorTemp : Inport  Port=2
  Bus Creator : BusCreator  Inputs=2
  MotorLowerTempDiag : Subsystem
  MotorOverTempDiag : Subsystem
  MotorTempFltInfo : Outport
  wires:
  SysSelfCheckDownFlg/1 -> MotorLowerTempDiag/1(SysSelfCheckDownFlg), MotorOverTempDiag/1(SysSelfCheckDownFlg)
  MotorTemp/1 -> MotorLowerTempDiag/2(MotorTemp), MotorOverTempDiag/2(MotorTemp)
  MotorOverTempDiag/1(MotorOverTempFltInfo) -> Bus Creator/1  "MotorOverTempFltInfo"
  MotorLowerTempDiag/1(MotorLowerTempFltInfo) -> Bus Creator/2  "MotorLowerTempFltInfo"
  Bus Creator/1 -> MotorTempFltInfo/1

== system FaultCheck/FaultDiagnose/PCBTempDiag ==
  SysSelfCheckDownFlg : Inport
  PCBTemp : Inport  Port=2
  Bus Creator : BusCreator  Inputs=2
  PCBLowerTempDiag : Subsystem
  PCBOverTempDiag : Subsystem
  PCBTempFltInfo : Outport
  wires:
  Bus Creator/1 -> PCBTempFltInfo/1
  PCBLowerTempDiag/1(PCBLowerTempFltInfo) -> Bus Creator/2  "PCBLowerTempFltInfo"
  SysSelfCheckDownFlg/1 -> PCBLowerTempDiag/1(SysSelfCheckDownFlg), PCBOverTempDiag/1(SysSelfCheckDownFlg)
  PCBTemp/1 -> PCBLowerTempDiag/2(PCBTemp), PCBOverTempDiag/2(PCBTemp)
  PCBOverTempDiag/1(PCBOverTempFltInfo) -> Bus Creator/1  "PCBOverTempFltInfo"

== system FaultCheck/FaultDiagnose/PhaseCurrDiag ==
  SysSelfCheckDownFlg : Inport
  UPhaseCurr_A : Inport  Port=2
  VPhaseCurr_A : Inport  Port=3
  WPhaseCurr_A : Inport  Port=4
  Bus Creator : BusCreator  Inputs=3
  Flt_IuOverCurrDiag : Subsystem  TreatAsAtomicUnit=on
      settings: RTWSystemCode=Inline
  Flt_IvOverCurrDiag : Subsystem  TreatAsAtomicUnit=on
      settings: RTWSystemCode=Inline
  Flt_IwOverCurrDiag : Subsystem  TreatAsAtomicUnit=on
      settings: RTWSystemCode=Inline
  PhaseCurrOCFltInfo : Outport
  wires:
  UPhaseCurr_A/1 -> Flt_IuOverCurrDiag/2(UPhaseCurr_A)
  SysSelfCheckDownFlg/1 -> Flt_IuOverCurrDiag/1(SysSelfCheckDownFlg), Flt_IwOverCurrDiag/1(SysSelfCheckDownFlg), Flt_IvOverCurrDiag/1(SysSelfCheckDownFlg)
  VPhaseCurr_A/1 -> Flt_IvOverCurrDiag/2(VPhaseCurr_A)
  WPhaseCurr_A/1 -> Flt_IwOverCurrDiag/2(WPhaseCurr_A)
  Flt_IvOverCurrDiag/1(IvOverCurrFltInfoOut) -> Bus Creator/2  "IvOverCurrFltInfoOut"
  Flt_IuOverCurrDiag/1(IuOverCurrFltInfoOut) -> Bus Creator/1  "IuOverCurrFltInfoOut"
  Flt_IwOverCurrDiag/1(IwOverCurrFltInfoOut) -> Bus Creator/3  "IwOverCurrFltInfoOut"
  Bus Creator/1 -> PhaseCurrOCFltInfo/1

== system FaultCheck/FaultDiagnose/UdcLowerOneDiag ==
  SysSelfCheckDownFlg : Inport
  Udc : Inport  Port=2
  Bus Creator : BusCreator  Inputs=3
  Bus Selector : BusSelector  OutputSignals=UdcLowerOneDiagEn
  Bus Selector1 : BusSelector  OutputSignals=UdcLowerOneFltLevel,UdcLowerOnePowerCoeff
  Diagnose : Subsystem
  EnableJudgement : Subsystem
  FaultLevelDeter : Subsystem
  Parameters : Subsystem
  PowerReductionCoeffDeter : Subsystem
  UdcLowerOneInfo : Outport
  wires:
  Udc/1 -> Diagnose/2(Udc), Parameters/1(Udc)
  SysSelfCheckDownFlg/1 -> EnableJudgement/1(SysSelfCheckDownFlg)
  Parameters/1(Param) -> Diagnose/3(Parameter), Bus Selector1/1, Bus Selector/1
  Bus Selector/1 -> EnableJudgement/2(DiagEn)  "<UdcLowerOneDiagEn>"
  EnableJudgement/1(DiagEnOut) -> Diagnose/1(DiagEnOut)
  Bus Selector1/2 -> PowerReductionCoeffDeter/2(PowerCoeff)  "<UdcLowerOnePowerCoeff>"
  FaultLevelDeter/1(UdcLowerOneFltLevelOut) -> Bus Creator/2, PowerReductionCoeffDeter/1(UdcLowerOneFltLevelOut)  "UdcLowerOneFltLevelOut"
  Diagnose/1(UdcLowerOneFlgOut) -> Bus Creator/1, FaultLevelDeter/1(UdcLowerOneFlgOut)  "UdcLowerOneFlgOut"
  PowerReductionCoeffDeter/1(UdcLowerOnePowerCoeffOut) -> Bus Creator/3  "UdcLowerOnePowerCoeffOut"
  Bus Selector1/1 -> FaultLevelDeter/2(FaultLevel)  "<UdcLowerOneFltLevel>"
  Bus Creator/1 -> UdcLowerOneInfo/1

== system FaultCheck/FaultDiagnose/UdcLowerTwoDiag ==
  SysSelfCheckDownFlg : Inport
  Udc : Inport  Port=2
  Bus Creator : BusCreator  Inputs=3
  Bus Selector : BusSelector  OutputSignals=UdcLowerTwoDiagEn
  Bus Selector1 : BusSelector  OutputSignals=UdcLowerTwoFltLevel,UdcLowerTwoPowerCoeff
  Diagnose : Subsystem
  EnableJudgement : Subsystem
  FaultLevelDeter : Subsystem
  Parameters : Subsystem
  PowerReductionCoeffDeter : Subsystem
  UdcLowerTwoInfo : Outport
  wires:
  FaultLevelDeter/1(UdcLowerTwoFltLevelOut) -> Bus Creator/2, PowerReductionCoeffDeter/1(UdcLowerTwoFltLevelOut)  "UdcLowerTwoFltLevelOut"
  Bus Selector1/2 -> PowerReductionCoeffDeter/2(PowerCoeff)  "<UdcLowerTwoPowerCoeff>"
  EnableJudgement/1(DiagEnOut) -> Diagnose/1(DiagEnOut)
  Bus Selector1/1 -> FaultLevelDeter/2(FaultLevel)  "<UdcLowerTwoFltLevel>"
  Diagnose/1(UdcLowerTwoFlgOut) -> Bus Creator/1, FaultLevelDeter/1(UdcLowerTwoFlgOut)  "UdcLowerTwoFlgOut"
  Bus Selector/1 -> EnableJudgement/2(DiagEn)  "<UdcLowerTwoDiagEn>"
  Udc/1 -> Diagnose/2(Udc)
  PowerReductionCoeffDeter/1(UdcLowerTwoPowerCoeffOut) -> Bus Creator/3  "UdcLowerTwoPowerCoeffOut"
  Parameters/1(Param) -> Diagnose/3(Parameter), Bus Selector1/1, Bus Selector/1
  SysSelfCheckDownFlg/1 -> EnableJudgement/1(SysSelfCheckDownFlg)
  Bus Creator/1 -> UdcLowerTwoInfo/1

== system FaultCheck/FaultDiagnose/UdcOverOneDiag ==
  SysSelfCheckDownFlg : Inport
  Udc : Inport  Port=2
  Bus Creator : BusCreator  Inputs=3
  Bus Selector : BusSelector  OutputSignals=UdcOverOneDiagEn
  Bus Selector1 : BusSelector  OutputSignals=UdcOverOneFltLevel
  Bus Selector2 : BusSelector  OutputSignals=UdcOverOnePowerCoeff
  Diagnose : Subsystem
  EnableJudgement : Subsystem
  FaultLevelDeter : Subsystem
  Parameter : Subsystem
  PowerReductionCoeffDeter : Subsystem
  UdcOverOneFltInfo : Outport
  wires:
  SysSelfCheckDownFlg/1 -> EnableJudgement/1(SysSelfCheckDownFlg)
  Udc/1 -> Diagnose/2(Udc), Parameter/1(Udc)
  Bus Selector/1 -> EnableJudgement/2(DiagEn)  "<UdcOverOneDiagEn>"
  EnableJudgement/1(DiagEnOut) -> Diagnose/1(DiagEnOut)
  FaultLevelDeter/1(UdcOverOneFltLevelOut) -> Bus Creator/2, PowerReductionCoeffDeter/1(UdcOverOneFltLevelOut)  "UdcOverOneFltLevelOut"
  Diagnose/1(UdcOverOneFlgOut) -> Bus Creator/1, FaultLevelDeter/1(UdcOverOneFlgOut)  "UdcOverOneFlgOut"
  Bus Selector1/1 -> FaultLevelDeter/2(FaultLevel)  "<UdcOverOneFltLevel>"
  Parameter/1(Parameter) -> Diagnose/3(Parameter), Bus Selector1/1, Bus Selector2/1, Bus Selector/1
  Bus Selector2/1 -> PowerReductionCoeffDeter/2(PowerCoeff)  "<UdcOverOnePowerCoeff>"
  PowerReductionCoeffDeter/1(UdcOverOnePowerCoeffOut) -> Bus Creator/3  "UdcOverOnePowerCoeffOut"
  Bus Creator/1 -> UdcOverOneFltInfo/1

== system FaultCheck/FaultDiagnose/UdcOverTwoDiag ==
  SysSelfCheckDownFlg : Inport
  Udc : Inport  Port=2
  Bus Creator : BusCreator  Inputs=3
  Bus Selector : BusSelector  OutputSignals=UdcOverTwoDiagEn
  Bus Selector1 : BusSelector  OutputSignals=UdcOverTwoFltLevel
  Bus Selector2 : BusSelector  OutputSignals=UdcOverTwoPowerCoeff
  Diagnose : Subsystem
  EnableJudgement : Subsystem
  FaultLevelDeter : Subsystem
  Parameter : Subsystem
  PowerReductionCoeffDeter : Subsystem
  UdcOverTwoFltInfo : Outport
  wires:
  Bus Creator/1 -> UdcOverTwoFltInfo/1
  Bus Selector1/1 -> FaultLevelDeter/2(FaultLevel)  "<UdcOverTwoFltLevel>"
  PowerReductionCoeffDeter/1(UdcOverTwoPowerCoeffOut) -> Bus Creator/3  "UdcOverTwoPowerCoeffOut"
  EnableJudgement/1(DiagEnOut) -> Diagnose/1(DiagEnOut)
  FaultLevelDeter/1(UdcOverTwoFltLevelOut) -> Bus Creator/2, PowerReductionCoeffDeter/1(UdcOverTwoFltLevelOut)  "UdcOverTwoFltLevelOut"
  Bus Selector2/1 -> PowerReductionCoeffDeter/2(PowerCoeff)  "<UdcOverTwoPowerCoeff>"
  Parameter/1(Parameter) -> Diagnose/3(Parameter), Bus Selector1/1, Bus Selector2/1, Bus Selector/1
  Diagnose/1(UdcOverTwoFlgOut) -> Bus Creator/1, FaultLevelDeter/1(UdcOverTwoFlgOut)  "UdcOverTwoFlgOut"
  Bus Selector/1 -> EnableJudgement/2(DiagEn)  "<UdcOverTwoDiagEn>"
  SysSelfCheckDownFlg/1 -> EnableJudgement/1(SysSelfCheckDownFlg)
  Udc/1 -> Diagnose/2(Udc)

== system FaultCheck/FltCheck/Determination ==
  FltSrc : Inport
  FltTh : Inport  Port=2
  Condition : Inport  Port=3
  ConfirmTh : Inport  Port=4
  ClearTh : Inport  Port=5
  FastRecover_one : Inport  Port=6
  Enable : EnablePort
  Detection Criteria : Subsystem
  Hysteresis : Subsystem
  FltConfirmed : Outport  OutputWhenDisabled=reset  InitialOutput=false
  wires:
  Detection Criteria/1(Fail) -> Hysteresis/1(Fail)
  ClearTh/1 -> Hysteresis/3(ClearTh)
  ConfirmTh/1 -> Hysteresis/2(ConfirmTh)
  Hysteresis/1(Out) -> FltConfirmed/1
  FastRecover_one/1 -> Hysteresis/4(FastRecover_one)
  FltSrc/1 -> Detection Criteria/1(FltSrc)
  FltTh/1 -> Detection Criteria/2(FltTh)
  Condition/1 -> Detection Criteria/3(Condition)

== system FaultCheck/LowerDelay/Hysteresis ==
  Fail : Inport
  ConfirmTh : Inport  Port=2
  ClearTh : Inport  Port=3
  FastRecover_one : Inport  Port=4
  Hysteresis_Chart : Stateflow chart  TreatAsAtomicUnit=on
  Out : Outport
  wires:
  Hysteresis_Chart/1(Out) -> Out/1
  FastRecover_one/1 -> Hysteresis_Chart/4(FastRecover_one)
  ConfirmTh/1 -> Hysteresis_Chart/3(ConfirmTh)
  ClearTh/1 -> Hysteresis_Chart/2(ClearTh)
  Fail/1 -> Hysteresis_Chart/1(Fail)

== system FaultCheck/LowerDelay/Relay ==
  FltSrc : Inport
  FltTh : Inport  Port=2
  RecoverFltTh : Inport  Port=3
  Data Type Conversion : DataTypeConversion  OutDataTypeStr=boolean  SaturateOnIntegerOverflow=off  RndMeth=Floor
  Relay_Chart : Stateflow chart  TreatAsAtomicUnit=on
      settings: PortSchema="{\"entries\":[{\"content\":{\"sides\":[{\"content\":{\"connectorIds\":[\"In2\",\"In3\",\"In1\",\"In4\"]},\"type\":\"ConnectorPlacement.EquallySpacedRectSide\",\"uuid\":\"134e3c61-5d02-4b29-842b-11374aeafb34\"},{\"content\":{\"connectorIds\":[\"Out1\"],\"side\":\"RIGHT\"},\"type\":\"ConnectorPlacement.EquallySpacedRectSide\",\"uuid\":\"4da8ce31-3f03-4a1a-80ea-9a46854268ed\"},{\"content\":{\"connectorIds\":[],\"side\":\"TOP\"},\"type\":\"ConnectorPlacement.EquallySpacedRectSide\",\"uuid\":\"177448d7-b001-4933-86b0-df440ef4cded\"},{\"content\":{\"connectorIds\":[],\"side\":\"BOTTOM\"},\"type\":\"ConnectorPlacement.EquallySpacedRectSide\",\"uuid\":\"d0ffd9ad-4245-4732-8afe-5f2e62e505b1\"}]},\"type\":\"ConnectorPlacement.EquallySpacedConnector\",\"uuid\":\"1e95b7e2-f21d-4f4c-bea9-13f973fc4e55\"}],\"packageUris\":[\"http://schema.mathworks.com/mf0/Connector/R2020b\"],\"version\":\"1.0\"}"
  Unit Delay : UnitDelay  SampleTime=-1  HasFrameUpgradeWarning=on
  Fail : Outport
  wires:
  Unit Delay/1 -> Relay_Chart/4(Faildelay)
  Data Type Conversion/1 -> Unit Delay/1, Fail/1
  Relay_Chart/1(Fail) -> Data Type Conversion/1
  RecoverFltTh/1 -> Relay_Chart/1(RecoverFltTh)
  FltTh/1 -> Relay_Chart/3(FltTh)
  FltSrc/1 -> Relay_Chart/2(FltSrc)

== system FaultCheck/OverDelay/Hysteresis ==
  Fail : Inport
  ConfirmTh : Inport  Port=2
  ClearTh : Inport  Port=3
  FastRecover_one : Inport  Port=4
  Hysteresis_Chart : Stateflow chart  TreatAsAtomicUnit=on
  Out : Outport
  wires:
  Fail/1 -> Hysteresis_Chart/1(Fail)
  ClearTh/1 -> Hysteresis_Chart/2(ClearTh)
  ConfirmTh/1 -> Hysteresis_Chart/3(ConfirmTh)
  FastRecover_one/1 -> Hysteresis_Chart/4(FastRecover_one)
  Hysteresis_Chart/1(Out) -> Out/1

== system FaultCheck/OverDelay/Relay ==
  FltSrc : Inport
  FltTh : Inport  Port=2
  RecoverFltTh : Inport  Port=3
  Data Type Conversion : DataTypeConversion  OutDataTypeStr=boolean  SaturateOnIntegerOverflow=off  RndMeth=Floor
  Relay_Chart : Stateflow chart  TreatAsAtomicUnit=on
      settings: PortSchema="{\"entries\":[{\"content\":{\"sides\":[{\"content\":{\"connectorIds\":[\"In2\",\"In3\",\"In1\",\"In4\"]},\"type\":\"ConnectorPlacement.EquallySpacedRectSide\",\"uuid\":\"134e3c61-5d02-4b29-842b-11374aeafb34\"},{\"content\":{\"connectorIds\":[\"Out1\"],\"side\":\"RIGHT\"},\"type\":\"ConnectorPlacement.EquallySpacedRectSide\",\"uuid\":\"4da8ce31-3f03-4a1a-80ea-9a46854268ed\"},{\"content\":{\"connectorIds\":[],\"side\":\"TOP\"},\"type\":\"ConnectorPlacement.EquallySpacedRectSide\",\"uuid\":\"177448d7-b001-4933-86b0-df440ef4cded\"},{\"content\":{\"connectorIds\":[],\"side\":\"BOTTOM\"},\"type\":\"ConnectorPlacement.EquallySpacedRectSide\",\"uuid\":\"d0ffd9ad-4245-4732-8afe-5f2e62e505b1\"}]},\"type\":\"ConnectorPlacement.EquallySpacedConnector\",\"uuid\":\"1e95b7e2-f21d-4f4c-bea9-13f973fc4e55\"}],\"packageUris\":[\"http://schema.mathworks.com/mf0/Connector/R2020b\"],\"version\":\"1.0\"}"
  Unit Delay : UnitDelay  SampleTime=-1  HasFrameUpgradeWarning=on
  Fail : Outport
  wires:
  FltSrc/1 -> Relay_Chart/2(FltSrc)
  FltTh/1 -> Relay_Chart/3(FltTh)
  RecoverFltTh/1 -> Relay_Chart/1(RecoverFltTh)
  Relay_Chart/1(Fail) -> Data Type Conversion/1
  Data Type Conversion/1 -> Fail/1, Unit Delay/1
  Unit Delay/1 -> Relay_Chart/4(Faildelay)

== system FaultCheck/FaultDiag_HighTask_100us/FltDetermine/FliLvlOut ==
  Flt_HighTaskFltLvlOut : Inport
  Flt_MiddTaskFltLvlOut : Inport  Port=2
  Flt_LowTaskFltLvlOut : Inport  Port=3
  Max : MinMax  Function=max  Inputs=3
  Flt_FltLvlOut : Outport
  wires:
  Max/1 -> Flt_FltLvlOut/1
  Flt_LowTaskFltLvlOut/1 -> Max/3
  Flt_HighTaskFltLvlOut/1 -> Max/1
  Flt_MiddTaskFltLvlOut/1 -> Max/2

== system FaultCheck/FaultDiag_HighTask_100us/FltDetermine/PowRecCoefOut ==
  Flt_HighTaskPowRecCoef : Inport
  Flt_MiddTaskPowRecCoef : Inport  Port=2
  Flt_LowTaskPowRecCoef : Inport  Port=3
  Max : MinMax  Inputs=3
  Flt_PowRecCoef : Outport
  wires:
  Max/1 -> Flt_PowRecCoef/1
  Flt_HighTaskPowRecCoef/1 -> Max/1
  Flt_LowTaskPowRecCoef/1 -> Max/3
  Flt_MiddTaskPowRecCoef/1 -> Max/2

== system FaultCheck/FaultDiag_HighTask_100us/FltDetermine/Subsystem1 ==
  Flt_FltLvlOut : Inport
  Compare To Constant : simulink/Logic and Bit Operations/Compare To Constant  relop=<=  const=FLTLVL_TWO  OutDataTypeStr=boolean
  Constant10 : Constant  Value=FLT_SAFTY
  Constant9 : Constant  Value=FLT_FOCCONTROL
  Switch4 : Switch  Criteria=u2 ~= 0  SaturateOnIntegerOverflow=off  InputSameDT=off
  Flt_SwtForFOC : Outport
  wires:
  Constant10/1 -> Switch4/3
  Constant9/1 -> Switch4/1
  Switch4/1 -> Flt_SwtForFOC/1
  Compare To Constant/1 -> Switch4/2
  Flt_FltLvlOut/1 -> Compare To Constant/1

== system FaultCheck/FaultDiag_HighTask_100us/FltDetn/CurrentSensorDetn ==
  Sys_SelfChkFishFlg : Inport
  Flt_CurrentSensorFlg : Inport  Port=2
  IPC_IuRaw_A : Inport  Port=3
  IPC_IvRaw_A : Inport  Port=4
  Bus Creator : BusCreator  Inputs=2
  Enable : Subsystem
  Flt_CurrentSensorDetn : Subsystem
  Parameter : Subsystem
  Flt_CurrentSensorDetnOut : Outport
  wires:
  IPC_IvRaw_A/1 -> Flt_CurrentSensorDetn/5(IPC_IvRaw_A)
  IPC_IuRaw_A/1 -> Flt_CurrentSensorDetn/4(IPC_IuRaw_A)
  Flt_CurrentSensorFlg/1 -> Flt_CurrentSensorDetn/1(InPutVal1)
  Bus Creator/1 -> Flt_CurrentSensorDetnOut/1
  Flt_CurrentSensorDetn/1(Flt_CurrentSensorFltLvl) -> Bus Creator/1
  Flt_CurrentSensorDetn/2(Flt_CurrentSensorPowRecCoefOut) -> Bus Creator/2
  Parameter/1(Para) -> Flt_CurrentSensorDetn/3(Para)
  Enable/1(Enable) -> Flt_CurrentSensorDetn/2(EnabDetn)
  Sys_SelfChkFishFlg/1 -> Enable/1(Sys_SelfChkFishFlg)

== system FaultCheck/FaultDiag_HighTask_100us/FltDetn/CurrentZeroDrfDetn ==
  note: Flt_CurrZeroDrf_ActvnErrDetn
      | Uint8
      | 电流零飘诊断使能标志位
      |
      | Flt_CurrZeroDrf_ErrCode
      | Uint16
      | 电流零飘故障码
  note: 故障诊断主体模块主要包括四个部分，故障诊断标志位判断、故障等级判断、降功率系数判断和故障码记录
      | 1、故障诊断标志位判断：根据使能标志位判断进入，最后确认其故障标志位的值
      | 2、故障码记录：根据故障标志位记录相关故障码，0还是标定量。
      | 3、故障等级判断：根据故障标志位确定相关故障等级，是0还是标定量
      | 4、降功率系数判断：根据故障等级进行判断选择对应的降功率系数
      |
      | 故障标志位的判断：
      | 当输入的电流零飘标志位为1，并持续标定的次数，故障标志位置1，否者保留上一时刻的故障标志位0，不可恢复。
      |
      | 由于电流零飘只做一次，进入诊断时将电流零飘记次，当电流零飘完成标志位置1且电流零飘记次为0时，才进行电流零飘的诊断
  CurrentReadingCaliFlag : Inport
  Enable1 : EnablePort
  Bus Creator : BusCreator  Inputs=2
  Constant : Constant  Value=CurrZeroDrfDetn_Counter  OutDataTypeStr=uint8
  CurrZeroDrfDetn : Subsystem
  Enable : Subsystem
  Parameter : Subsystem
  Unit Delay : UnitDelay  SampleTime=-1  HasFrameUpgradeWarning=on
  Flt_CurrZeroDrfDetn : Outport
  CurrZeroDrfDetnFlg : Outport  Port=2
  wires:
  CurrentReadingCaliFlag/1 -> CurrZeroDrfDetn/1(InPutVal)
  Enable/1(Enable) -> CurrZeroDrfDetn/2(EnabDetn)
  Bus Creator/1 -> Flt_CurrZeroDrfDetn/1
  CurrZeroDrfDetn/2(Flt_CurrZeroDrfPowRecCoefOut) -> Bus Creator/2
  Parameter/1(Para) -> CurrZeroDrfDetn/3(Para)
  CurrZeroDrfDetn/1(Flt_CurrZeroDrfFltLvl) -> Bus Creator/1
  Constant/1 -> Unit Delay/1
  Unit Delay/1 -> CurrZeroDrfDetnFlg/1

== system FaultCheck/FaultDiag_HighTask_100us/FltDetn/DriveUdcDetn ==
  note: Flt_DriveUdc_ErrDeb
      | Uint8
      | 驱动电压故障判断次数
      |
      | Flt_DriveUdc_ActvnDetn
      | Uint8
      | 驱动电压故障使能标志位
      |
      | Flt_DriveUdc_ErrCode
      | Uint16
      | 驱动电压故障码
  note: 故障诊断主体模块主要包括四个部分，故障诊断标志位判断、故障等级判断、降功率系数判断和故障码记录
      | 1、故障诊断标志位判断：根据使能标志位判断进入，最后确认其故障标志位的值
      | 2、故障码记录：根据故障标志位记录相关故障码，0还是标定量。
      | 3、故障等级判断：根据故障标志位确定相关故障等级，是0还是标定量
      | 4、降功率系数判断：根据故障等级进行判断选择对应的降功率系数
      |
      | 故障标志位的判断：
      | 当输入的驱动电压标志位为1，并持续标定的次数，故障标志位置1，否者保留上一时刻的故障标志位0，不可恢复。
  IPT_Drive_Udc_Error_Flg : Inport
  Sys_SelfChkFishFlg : Inport  Port=2
  Bus Creator : BusCreator  Inputs=2
  DriveUdcDetn : Subsystem
  Enable : Subsystem
  Parameter : Subsystem
  Flt_DriveUdcDetnOut : Outport
  wires:
  Enable/1(Enable) -> DriveUdcDetn/2(EnabDetn)
  DriveUdcDetn/1(Flt_DriveUdcFltLvl) -> Bus Creator/1
  DriveUdcDetn/2(Flt_DriveUdcPowRecCoefOut) -> Bus Creator/2
  Parameter/1(Para) -> DriveUdcDetn/3(Para)
  Bus Creator/1 -> Flt_DriveUdcDetnOut/1
  IPT_Drive_Udc_Error_Flg/1 -> DriveUdcDetn/1(InPutVal1)
  Sys_SelfChkFishFlg/1 -> Enable/1(Sys_SelfChkFishFlg)

== system FaultCheck/FaultDiag_HighTask_100us/FltDetn/Drive_H_Detn ==
  note: Flt_Drive_H_ErrDeb
      | Uint8
      | 驱动上桥故障判断次数
      |
      | Flt_Drive_H_ActvnDetn
      | Uint8
      | 驱动上桥故障使能标志位
      |
      | Flt_Drive_H_ErrCode
      | Uint16
      | 驱动上桥故障码
  note: 故障诊断主体模块主要包括四个部分，故障诊断标志位判断、故障等级判断、降功率系数判断和故障码记录
      | 1、故障诊断标志位判断：根据使能标志位判断进入，最后确认其故障标志位的值
      | 2、故障码记录：根据故障标志位记录相关故障码，0还是标定量。
      | 3、故障等级判断：根据故障标志位确定相关故障等级，是0还是标定量
      | 4、降功率系数判断：根据故障等级进行判断选择对应的降功率系数
      |
      | 故障标志位的判断：
      | 当输入的驱动上桥故障标志位标志位为1，并持续标定的次数，故障标志位置1，否者保留上一时刻的故障标志位0，不可恢复。
  IPT_Hw_EDI_H_Error_Flg : Inport
  Sys_SelfChkFishFlg : Inport  Port=2
  Bus Creator : BusCreator  Inputs=2
  Drive_H_Detn : Subsystem
  Enable : Subsystem
  Parameter : Subsystem
  Flt_Drive_H_DetnOut : Outport
  wires:
  Enable/1(Enable) -> Drive_H_Detn/2(EnabDetn)
  Drive_H_Detn/1(Flt_Drive_H_FltLvl) -> Bus Creator/1
  Drive_H_Detn/2(Flt_Drive_H_PowRecCoefOut) -> Bus Creator/2
  Parameter/1(Para) -> Drive_H_Detn/3(Para)
  Bus Creator/1 -> Flt_Drive_H_DetnOut/1
  IPT_Hw_EDI_H_Error_Flg/1 -> Drive_H_Detn/1(InPutVal1)
  Sys_SelfChkFishFlg/1 -> Enable/1(Sys_SelfChkFishFlg)

== system FaultCheck/FaultDiag_HighTask_100us/FltDetn/Drive_L_Detn ==
  note: Flt_Drive_L_ErrDeb
      | Uint8
      | 驱动下桥故障判断次数
      |
      | Flt_Drive_L_ActvnDetn
      | Uint8
      | 驱动下桥故障使能标志位
      |
      | Flt_Drive_L_ErrCode
      | Uint16
      | 驱动下桥故障码
  note: 故障诊断主体模块主要包括四个部分，故障诊断标志位判断、故障等级判断、降功率系数判断和故障码记录
      | 1、故障诊断标志位判断：根据使能标志位判断进入，最后确认其故障标志位的值
      | 2、故障码记录：根据故障标志位记录相关故障码，0还是标定量。
      | 3、故障等级判断：根据故障标志位确定相关故障等级，是0还是标定量
      | 4、降功率系数判断：根据故障等级进行判断选择对应的降功率系数
      |
      | 故障标志位的判断：
      | 当输入的驱动下桥故障标志位标志位为1，并持续标定的次数，故障标志位置1，否者保留上一时刻的故障标志位0，不可恢复。
  IPT_Hw_EDI_L_Error_Flg : Inport
  Sys_SelfChkFishFlg : Inport  Port=2
  Bus Creator : BusCreator  Inputs=2
  Drive_L_Detn : Subsystem
  Enable : Subsystem
  Parameter : Subsystem
  Flt_Drive_L_DetnOut : Outport
  wires:
  Enable/1(Enable) -> Drive_L_Detn/2(EnabDetn)
  Drive_L_Detn/1(Flt_Drive_L_FltLvl) -> Bus Creator/1
  Drive_L_Detn/2(Flt_Drive_L_PowRecCoefOut) -> Bus Creator/2
  Parameter/1(Para) -> Drive_L_Detn/3(Para)
  Bus Creator/1 -> Flt_Drive_L_DetnOut/1
  IPT_Hw_EDI_L_Error_Flg/1 -> Drive_L_Detn/1(InPutVal1)
  Sys_SelfChkFishFlg/1 -> Enable/1(Sys_SelfChkFishFlg)

== system FaultCheck/FaultDiag_HighTask_100us/FltDetn/HWOverCurrDetn ==
  note: Flt_HWOverCurr_ErrDeb
      | Uint8
      | 硬件过流诊断判断次数
      |
      | Flt_HWOverCurr_ActvnDetn
      | Uint8
      | 硬件过流诊断使能标志位
      |
      | Flt_HWOverCurr_ErrCode
      | Uint16
      | 硬件过流故障码
      |
      | Flt_CurrZeroDrf_ActvnErrDetn
      | Uint8
      | 电流零飘诊断使能标志位
      |
      | Flt_CurrZeroDrf_ErrCode
      | Uint16
      | 电流零飘故障码
  note: 故障诊断主体模块主要包括四个部分，故障诊断标志位判断、故障等级判断、降功率系数判断和故障码记录
      | 1、故障诊断标志位判断：根据使能标志位判断进入，最后确认其故障标志位的值
      | 2、故障码记录：根据故障标志位记录相关故障码，0还是标定量。
      | 3、故障等级判断：根据故障标志位确定相关故障等级，是0还是标定量
      | 4、降功率系数判断：根据故障等级进行判断选择对应的降功率系数
      |
      | 故障标志位的判断：
      | 当输入的硬件过流标志位为1，并持续标定的次数，故障标志位置1，否者保留上一时刻的故障标志位0，不可恢复。
  IPT_HWOverCurrRaw : Inport
  Sys_SelfChkFishFlg : Inport  Port=2
  Bus Creator : BusCreator  Inputs=2
  Enable : Subsystem
  HWOverCurrDetn : Subsystem
  Parameter : Subsystem
  Flt_HWOverCurrDetnOut : Outport
  wires:
  Enable/1(Enable) -> HWOverCurrDetn/2(EnabDetn)
  HWOverCurrDetn/1(Flt_HWOverCurrFltLvl) -> Bus Creator/1
  HWOverCurrDetn/2(Flt_HWOverCurrPowRecCoefOut) -> Bus Creator/2
  Parameter/1(Para) -> HWOverCurrDetn/3(Para)
  Bus Creator/1 -> Flt_HWOverCurrDetnOut/1
  IPT_HWOverCurrRaw/1 -> HWOverCurrDetn/1(InPutVal1)
  Sys_SelfChkFishFlg/1 -> Enable/1(Sys_SelfChkFishFlg)

== system FaultCheck/FaultDiag_HighTask_100us/FltDetn/HWOverUdcDetn ==
  note: Flt_HWOverUdc_ErrDeb
      | Uint8
      | 硬件过压判断次数
      |
      | Flt_HWOverUdc_ActvnDetn
      | Uint8
      | 硬件过压使能标志位
      |
      | Flt_HWOverUdc_ErrCode
      | Uint16
      | 硬件过压故障码
  note: 故障诊断主体模块主要包括四个部分，故障诊断标志位判断、故障等级判断、降功率系数判断和故障码记录
      | 1、故障诊断标志位判断：根据使能标志位判断进入，最后确认其故障标志位的值
      | 2、故障码记录：根据故障标志位记录相关故障码，0还是标定量。
      | 3、故障等级判断：根据故障标志位确定相关故障等级，是0还是标定量
      | 4、降功率系数判断：根据故障等级进行判断选择对应的降功率系数
      |
      | 故障标志位的判断：
      | 当输入的硬件过压标志位为1，并持续标定的次数，故障标志位置1，否者保留上一时刻的故障标志位0，不可恢复。
  IPT_Hw_DCLINK_OV_Error_Flg : Inport
  Sys_SelfChkFishFlg : Inport  Port=2
  Bus Creator : BusCreator  Inputs=2
  Enable : Subsystem
  HWOverCurrDetn : Subsystem
  Parameter : Subsystem
  Flt_HWOverCurrDetnOut : Outport
  wires:
  Enable/1(Enable) -> HWOverCurrDetn/2(EnabDetn)
  HWOverCurrDetn/1(Flt_HWOverUdcFltLvl) -> Bus Creator/1
  HWOverCurrDetn/2(Flt_HWOverUdcPowRecCoefOut) -> Bus Creator/2
  Parameter/1(Para) -> HWOverCurrDetn/3(Para)
  Bus Creator/1 -> Flt_HWOverCurrDetnOut/1
  IPT_Hw_DCLINK_OV_Error_Flg/1 -> HWOverCurrDetn/1(InPutVal1)
  Sys_SelfChkFishFlg/1 -> Enable/1(Sys_SelfChkFishFlg)

== system FaultCheck/FaultDiag_HighTask_100us/FltDetn/OverCurrDetn ==
  note: 序号
      | 变量名
      | 数据类型
      | 说明
      |
      | 1
      | Flt_IuOverCurr_HiLimPositv
      | single
      | u相过流的正向阈值
      |
      | 2
      | Flt_IuOverCurr_HiLimNegatv
      | single
      | u相过流的负向阈值
      |
      | 3
      | Flt_IuOverCurr_ErrDeb
      | Uint8
      | u相过流诊断判断次数
      |
      | 4
      | Flt_IuOverCurr_ActvErrDetn
      | Uint8
      | u相过流诊断使能标志位
      |
      | 5
      | Flt_IuOverCurr_ErrCode
      | Uint16
      | u相过流故障码
      |
      | 6
      | Flt_IvOverCurr_HiLimPositv
      | single
      | v相过流的正向阈值
      |
      | 7
      | Flt_IvOverCurr_HiLimNegatv
      | single
      | v相过流的负向阈值
      |
      | 8
      | Flt_IvOverCurr_ErrDeb
      | Uint8
      | v相过流诊断判断次数
      |
      | 9
      | Flt_IvOverCurr_ActvErrDetn
      | Uint8
      | v相过流诊断使能标志位
      |
      | 10
      | Flt_IvOverCurr_ErrCode
      | Uint16
      | v相过流故障码
      |
      | 11
      | Flt_IwOverCurr_HiLimPositv
      | single
      | w相过流的正向阈值
      |
      | 12
      | Flt_IwOverCurr_HiLimNegatv
      | single
      | w相过流的负向阈值
      |
      | 13
      | Flt_IwOverCurr_ErrDeb
      | Uint8
      | w相过流诊断判断次数
      |
      | 14
      | Flt_IwOverCurr_ActvErrDetn
      | Uint8
      | w相过流诊断使能标志位
      |
      | 15
      | Flt_IwOverCurr_ErrCode
      | Uint16
      | w相过流故障码
  note: 故障诊断主体模块主要包括四个部分，故障诊断标志位判断、故障等级判断、降功率系数判断和故障码记录
      | 1、故障诊断标志位判断：根据使能标志位判断进入，最后确认其故障标志位的值
      | 2、故障码记录：根据故障标志位记录相关故障码，0还是标定量。
      | 3、故障等级判断：根据故障标志位确定相关故障等级，是0还是标定量
      | 4、降功率系数判断：根据故障等级进行判断选择对应的降功率系数
      |
      | 故障标志位的判断：
      | 当输入电流大于电流正负阈值，并持续标定的次数，故障标志位置1，否者保留上一时刻的故障标志位，不可恢复。
  IPC_IuRaw_A : Inport
  IPC_IvRaw_A : Inport  Port=2
  IPC_IwRaw_A : Inport  Port=3
  Sys_SelfChkFishFlg : Inport  Port=4
  Bus Creator : BusCreator  Inputs=3
  Enable : Subsystem
  Flt_IuOverCurrDetn : Subsystem
  Flt_IvOverCurrDetn : Subsystem
  Flt_IwOverCurrDetn1 : Subsystem
  Parameter : Subsystem
  Parameter1 : Subsystem
  Parameter2 : Subsystem
  Flt_OverCurrDetnOut : Outport
  wires:
  Parameter/1(Para) -> Flt_IuOverCurrDetn/3(Para)
  Enable/1(Enable) -> [Enable], Flt_IuOverCurrDetn/2(EnabDetn)
  IPC_IuRaw_A/1 -> Flt_IuOverCurrDetn/1(InPutVal)
  Sys_SelfChkFishFlg/1 -> Enable/1(Sys_SelfChkFishFlg)
  Flt_IuOverCurrDetn/1(IuOverCurrDetnOut) -> Bus Creator/1  "Flt_IuOverCurrDetnOut"
  Bus Creator/1 -> Flt_OverCurrDetnOut/1
  IPC_IvRaw_A/1 -> Flt_IvOverCurrDetn/1(InPutVal)
  Parameter1/1(Para) -> Flt_IvOverCurrDetn/3(Para)
  [Enable] -> Flt_IvOverCurrDetn/2(EnabDetn)
  Flt_IvOverCurrDetn/1(IvOverCurrDetnOut) -> Bus Creator/2  "Flt_IvOverCurrDetnOut"
  Parameter2/1(Para) -> Flt_IwOverCurrDetn1/3(Para)
  Flt_IwOverCurrDetn1/1(IwOverCurrDetnOut) -> Bus Creator/3  "Flt_IwOverCurrDetnOut"
  IPC_IwRaw_A/1 -> Flt_IwOverCurrDetn1/1(InPutVal)
  [Enable] -> Flt_IwOverCurrDetn1/2(EnabDetn)
